simulink model "Plant_2_2"  (R2024b)
settings: Solver=VariableStepAuto  StartTime=0.0  StopTime=4  FixedStep=0.02  RelTol=1e-3
PreLoadFcn:
  | addpath("ref_source\2s\")
model workspace (MAT data in the model file):
  Ref_sig_idx = 2
values from neighbouring files (symbols this model uses):
  A = zeros(4, 4)    [Initialise_var_0.m]
  B = zeros(4, 2)    [Initialise_var_0.m]
  C = [1 0 0 0; 0 1 0 0; 0 0 1 0; 0 0 0 1]    [Initialise_var_0.m]    (also in leunberger_obs_1.m = [1 0 0 0; 0 1 0 0]; sfbia.m = [1 0 0 0; 0 1 0 0])
  D = [0 0; 0 0; 0 0; 0 0]    [Initialise_var_0.m]    (also in leunberger_obs_1.m = [0 0;0 0]; sfbia.m = [0 0;0 0])
  K = place(A, B, desired_poles)    [leunberger_obs_1.m]    (also in state_feedback.m; state_feedback_0.m; state_feedback_3.m; state_feedback_4.m = lqr(A,B,Q,R))
  K_r = -inv(inv(A-B*K)*B)    [state_feedback.m]    (also in state_feedback_0.m = -inv(E*inv(A-B*K)*B); state_feedback_3.m = -inv(E*inv(A-B*K)*B); state_feedback_4.m = -inv(E*inv(A-B*K)*B))
  L1 = 0.095    [Initialise_var_0.m]
  L2 = 0.095    [Initialise_var_0.m]
settings Model: Creator=Sez26  LastModifiedBy=Sez26

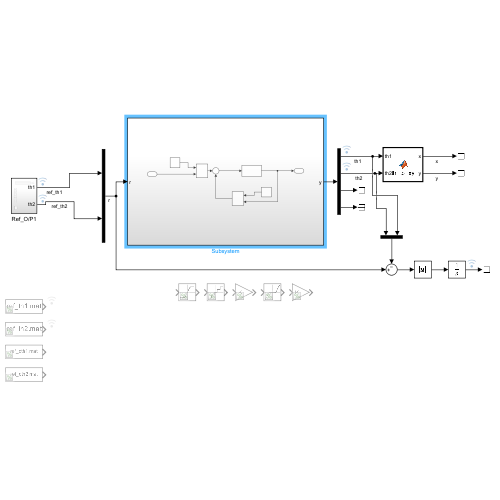
[thumbnail: Simulink's stored preview of the top-level diagram]
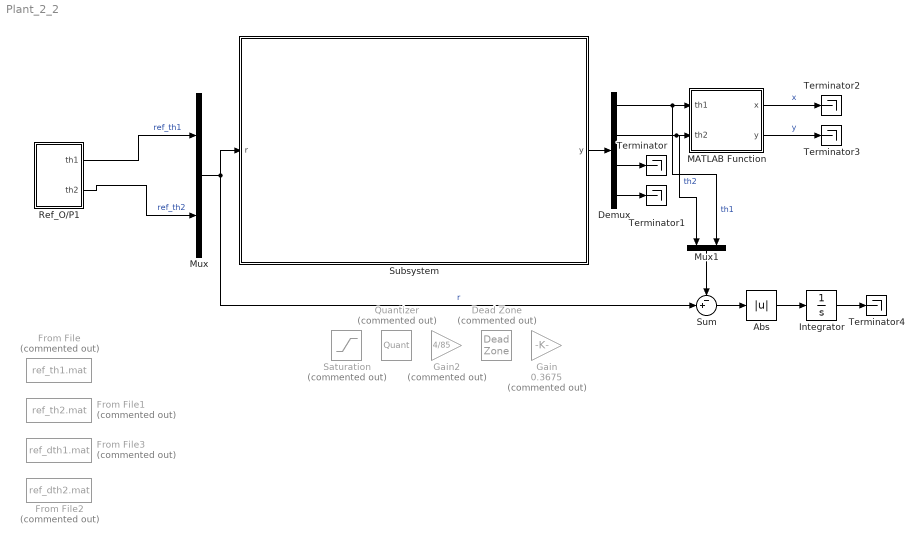
== system Plant_2_2 ==
  Abs : Abs  SaturateOnIntegerOverflow=off
  Dead Zone : DeadZone  Commented=on  LowerValue=-2.1  UpperValue=2.1
  Demux : Demux
  From File : FromFile  Commented=on  FileName=ref_th1.mat  SampleTime=0
  From File1 : FromFile  Commented=on  FileName=ref_th2.mat  SampleTime=0
  From File2 : FromFile  Commented=on  FileName=ref_dth2.mat  SampleTime=0
  From File3 : FromFile  Commented=on  FileName=ref_dth1.mat  SampleTime=0
  Gain : Gain  Commented=on  Gain=0.3675
  Gain2 : Gain  Commented=on  Gain=4/85
  Integrator : Integrator
  MATLAB Function : MATLAB Function  TreatAsAtomicUnit=on
  Mux : Mux  Inputs=2
  Mux1 : Mux  Inputs=2
  Quantizer : Quantizer  Commented=on  QuantizationInterval=1
  Ref_O/P1 : Subsystem
  Saturation : Saturate  Commented=on  UpperLimit=255  LowerLimit=-255
  Subsystem : Subsystem
  Sum : Sum  Inputs=-+|
  Terminator{,1..4} (5 alike) : Terminator
  wires:
  MATLAB Function/1(x) -> Terminator2/1  "x"
  MATLAB Function/2(y) -> Terminator3/1  "y"
  Demux/2 -> Mux1/1, MATLAB Function/2(th2)  "th2"
  Demux/1 -> Mux1/2, MATLAB Function/1(th1)  "th1"
  Ref_O/P1/1(th1) -> Mux/1  "ref_th1"
  Ref_O/P1/2(th2) -> Mux/2  "ref_th2"
  Demux/3 -> Terminator/1
  Demux/4 -> Terminator1/1
  Mux/1 -> Sum/2, Subsystem/1(r)  "r"
  Subsystem/1(y) -> Demux/1
  Integrator/1 -> Terminator4/1
  Abs/1 -> Integrator/1
  Sum/1 -> Abs/1
  Mux1/1 -> Sum/1

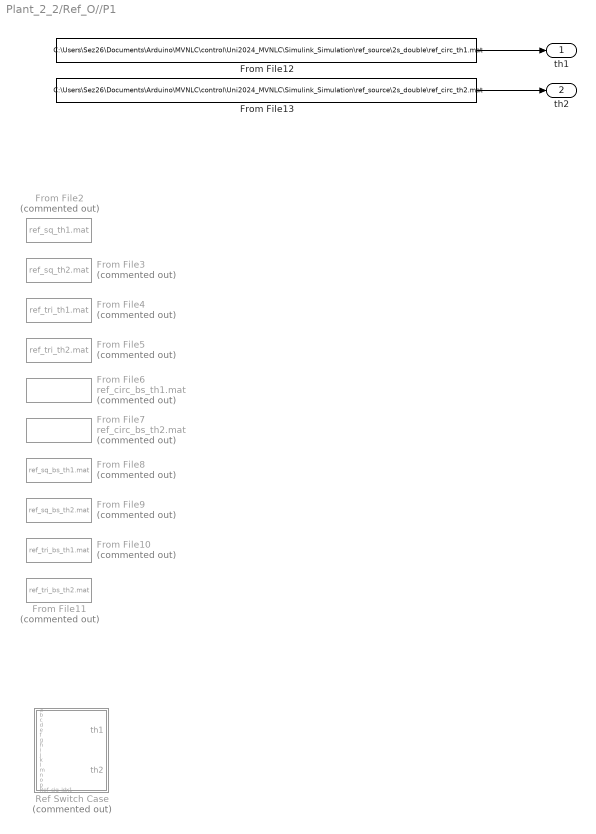
== system Plant_2_2/Ref_O//P1 ==
  From File10 : FromFile  Commented=on  FileName=ref_tri_bs_th1.mat  SampleTime=0
  From File11 : FromFile  Commented=on  FileName=ref_tri_bs_th2.mat  SampleTime=0
  From File12 : FromFile  FileName=C:\Users\Sez26\Documents\Arduino\MVNLC\control\Uni2024_MVNLC\Simulink_Simulation\ref_source\2s_double\ref_circ_th1.mat  SampleTime=0
  From File13 : FromFile  FileName=C:\Users\Sez26\Documents\Arduino\MVNLC\control\Uni2024_MVNLC\Simulink_Simulation\ref_source\2s_double\ref_circ_th2.mat  SampleTime=0
  From File2 : FromFile  Commented=on  FileName=ref_sq_th1.mat  SampleTime=0
  From File3 : FromFile  Commented=on  FileName=ref_sq_th2.mat  SampleTime=0
  From File4 : FromFile  Commented=on  FileName=ref_tri_th1.mat  SampleTime=0
  From File5 : FromFile  Commented=on  FileName=ref_tri_th2.mat  SampleTime=0
  From File6 : FromFile  Commented=on  FileName=ref_circ_bs_th1.mat  SampleTime=0
  From File7 : FromFile  Commented=on  FileName=ref_circ_bs_th2.mat  SampleTime=0
  From File8 : FromFile  Commented=on  FileName=ref_sq_bs_th1.mat  SampleTime=0
  From File9 : FromFile  Commented=on  FileName=ref_sq_bs_th2.mat  SampleTime=0
  Ref Switch Case : MATLAB Function  Commented=on  TreatAsAtomicUnit=on
  th1 : Outport
  th2 : Outport  Port=2
  wires:
  From File12/1 -> th1/1
  From File13/1 -> th2/1

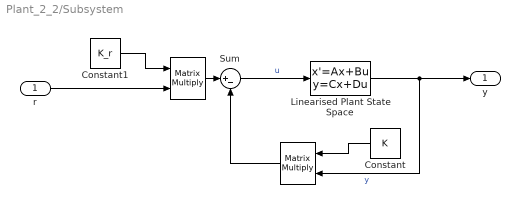
== system Plant_2_2/Subsystem ==
  r : Inport
  " " : Product  Multiplication=Matrix(*)
  "   " : Product  Multiplication=Matrix(*)
  Constant : Constant  Value=K
  Constant1 : Constant  Value=K_r
  Linearised Plant State Space : StateSpace  A=A  B=B  C=C  D=D  InitialCondition=[30, -30, 0 , 0]
  Sum : Sum  Inputs=|+-
  y : Outport
  wires:
  Sum/1 -> Linearised Plant State Space/1  "u"
  Constant/1 -> "   "/1
  Constant1/1 -> " "/1
  r/1 -> " "/2
  "   "/1 -> Sum/2
  " "/1 -> Sum/1
  Linearised Plant State Space/1 -> y/1, "   "/2  "y"

== matlab function Plant_2_2/MATLAB Function ==
  data: x output; th1 input; y output; th2 input; L1 parameter; L2 parameter
function [x,y] = th_to_xy(th1, th2, L1, L2)
    x = L1*cos(deg2rad(th1)) + L2*cos(deg2rad(th2));
    y = L1*sin(deg2rad(th1)) + L2*sin(deg2rad(th2));

== matlab function Plant_2_2/Ref_O//P1/Ref Switch Case ==
  data: Ref_sig_idx parameter; a input; b input; c input; d input; e input; f input; g input; h input; i input; j input; k input; l input; m input; n input; o input; p input; Ref_sig_idx1 input; th1 output; th2 output
function [th1, th2] = ref_switch(Ref_sig_idx, a, b, c, d, e, f, g, h, i, j, k, l, m, n, o, p, Ref_sig_idx1)
    if Ref_sig_idx == 0
        % circ base
        th1 = a;
        th2 = b;
    elseif Ref_sig_idx == 1
        % sq base
        th1 = c;
        th2 = d;
    elseif Ref_sig_idx == 2
        % tri base
        th1 = e;
        th2 = f;
    end
    if Ref_sig_idx == 3
        % circ b spline
        th1 = g;
        th2 = h;
    elseif Ref_sig_idx == 4
        % sq b spline
        th1 = i;
        th2 = j;
    elseif Ref_sig_idx == 5
        % tri b spline
        th1 = k;
        th2 = l;
    end
    if Ref_sig_idx == 6
        % sq corner sf
        th1 = m;
        th2 = n;
    elseif Ref_sig_idx == 7
        % tri corner sf
        th1 = o;
        th2 = p;
    else
        % invalid reference choice
        disp('Error invalid reference choice')
        th1 = 0;
        th2 = 0;
    end
